simulink model "Filter_Responses"  (R2021a)
settings: Solver=VariableStepAuto  StartTime=0.0  StopTime=3  RelTol=1e-3
libraries: spsCurrentMeasurementLib x4, spsSeriesRLCBranchLib x4, spsVoltageMeasurementLib x4, spsGroundLib x2, spsUniversalBridgeLib x1, spsThreePhaseProgrammableVoltageSourceLib x1, spspowerguiLib x1
settings Model: Creator=Dell  LastModifiedBy=Dell
settings SolverCC: ZeroCrossControl=DisableAll

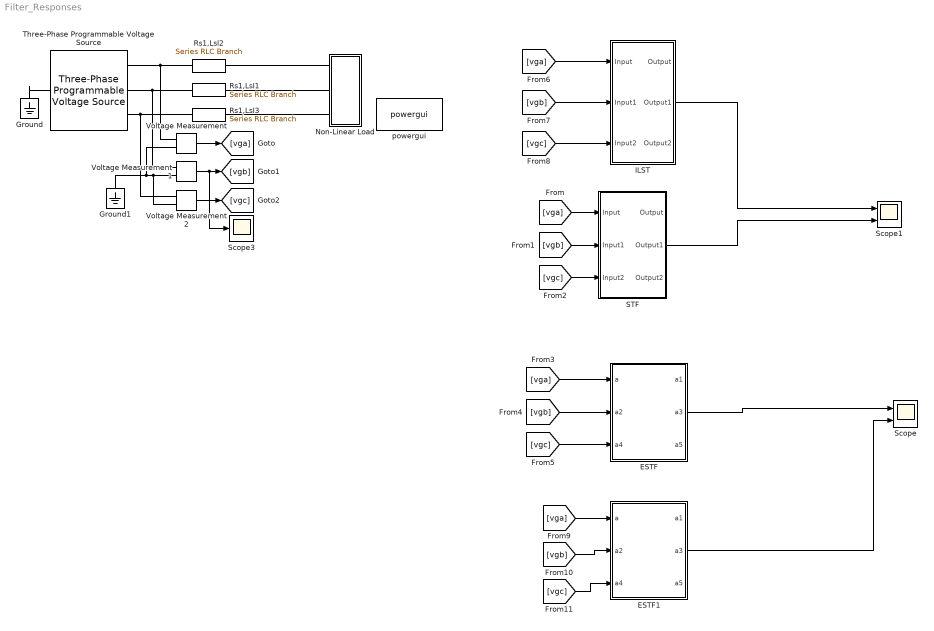
== system Filter_Responses ==
  ESTF : Subsystem
  ESTF1 : Subsystem
  Ground : spsGroundLib/Ground  LConnTagsString=a
  Ground1 : spsGroundLib/Ground  LConnTagsString=a
  ILST : Subsystem
  Non-Linear Load : Subsystem
  Rs1,LsI1 : spsSeriesRLCBranchLib/Series RLC Branch  LConnTagsString=__new0  RConnTagsString=__new0  BranchType=RL  Resistance=.1  Inductance=0.5e-3  SetiL0=off  InitialCurrent=0  Capacitance=1e-6  Setx0=off  InitialVoltage=0  Measurements=None
  Rs1,LsI2 : spsSeriesRLCBranchLib/Series RLC Branch  LConnTagsString=__new0  RConnTagsString=__new0  BranchType=RL  Resistance=.1  Inductance=0.5e-3  SetiL0=off  InitialCurrent=0  Capacitance=1e-6  Setx0=off  InitialVoltage=0  Measurements=None
  Rs1,LsI3 : spsSeriesRLCBranchLib/Series RLC Branch  LConnTagsString=__new0  RConnTagsString=__new0  BranchType=RL  Resistance=.1  Inductance=0.5e-3  SetiL0=off  InitialCurrent=0  Capacitance=1e-6  Setx0=off  InitialVoltage=0  Measurements=None
  STF : Subsystem
  Scope : Scope  NumInputPorts=2
  Scope1 : Scope  NumInputPorts=2
  Scope3 : Scope
  Three-Phase Programmable Voltage Source : spsThreePhaseProgrammableVoltageSourceLib/Three-Phase Programmable Voltage Source  PositiveSequence="[400  0 50]"  VariationEntity=None  VariationType=Table of time-amplitude pairs  VariationTypeAlt=Step  VariationStep=0.5  VariationRate=10  VariationMagnitude=0.3  VariationFrequency=2  VariationTiming=[1 2]  VariationPhaseA=off  Amplitudes=[1 0.8 1.2 1.0]  TimeValues=[0 0.1 0.15 0.2]  HarmonicGeneration=on  HarmonicA=[3 0.02 -25 0]  HarmonicB=[5 0.03 35 2]  Timing="[0.05  3]"  BusType=swing  Pref=0  Qref=0  Qmin=-inf  Qmax=inf
  Voltage Measurement : spsVoltageMeasurementLib/Voltage Measurement  PhasorSimulation=off  OutputType=Complex  PSBequivalent=0
  Voltage Measurement1 : spsVoltageMeasurementLib/Voltage Measurement  PhasorSimulation=off  OutputType=Complex  PSBequivalent=0
  Voltage Measurement2 : spsVoltageMeasurementLib/Voltage Measurement  PhasorSimulation=off  OutputType=Complex  PSBequivalent=0
  powergui : spspowerguiLib/powergui  Priority=1  SimulationMode=Discrete  SampleTime=5e-6  frequency=60  Iterations=50  frequencyindice=50  Pbase=100e6  ErrMax=1e-4  UnitsV=kV  UnitsW=MW  buscounter=0  FunctionMessages=off  echomessages=off  EnableUseOfTLC=off  CurrentSourceSwitches=off  DisableSnubberDevices=off  DisableRonSwitches=off  DisableVfSwitches=off  DisplayEquations=off  AutomaticDiscreteSolvers=off  SolverType=Tustin/Backward Euler (TBE)  Interpol=off  ExternalGateDelay=off  methode=off  Ts=100  x0status=blocks  SPID=on  SwTol=0  HookPort=off  NonlinearTolerance=1e-4  nMaxIteration=100  ContinueOnMaxIteration=off  RestoreLinks=warning  ResistiveCurrentMeasurement=off  Frange=[0:2:500]  Ylog=off  Xlog=on  ShowGrid=off  save=off  variable=ZData  structure=0  ZoomFFT=off  StartTime=0.0  cycles=1  DisplayStyle=1  fundamental=60  FreqAxis=off  MaxFrequency=1000  frequencyindicesteady=1  RmsSteady=1  display=off
  wires:
  Voltage Measurement/1 -> [vga]
  Voltage Measurement1/1 -> Scope3/1, [vgb]
  Voltage Measurement2/1 -> [vgc]
  [vga] -> STF/1(Input)
  [vgb] -> STF/2(Input1)
  [vgc] -> STF/3(Input2)
  [vgc] -> ESTF/3(a4)
  [vga] -> ESTF/1(a)
  [vgb] -> ESTF/2(a2)
  [vgc] -> ILST/3(Input2)
  [vga] -> ILST/1(Input)
  [vgb] -> ILST/2(Input1)
  ILST/2(Output1) -> Scope1/1
  STF/2(Output1) -> Scope1/2
  ESTF/2(a3) -> Scope/1
  [vga] -> ESTF1/1(a)
  [vgb] -> ESTF1/2(a2)
  [vgc] -> ESTF1/3(a4)
  ESTF1/2(a3) -> Scope/2
  connections:
  Three-Phase Programmable Voltage Source/RConn3 -- Voltage Measurement2/LConn1 -- Rs1,LsI3/LConn1
  Rs1,LsI1/LConn1 -- Voltage Measurement1/LConn1 -- Three-Phase Programmable Voltage Source/RConn2
  Rs1,LsI2/LConn1 -- Voltage Measurement/LConn1 -- Three-Phase Programmable Voltage Source/RConn1
  Rs1,LsI2/RConn1 -- Non-Linear Load/LConn1
  Rs1,LsI1/RConn1 -- Non-Linear Load/LConn2
  Rs1,LsI3/RConn1 -- Non-Linear Load/LConn3
  Ground/LConn1 -- Three-Phase Programmable Voltage Source/LConn1
  Ground1/LConn1 -- Voltage Measurement2/LConn2 -- Voltage Measurement1/LConn2 -- Voltage Measurement/LConn2

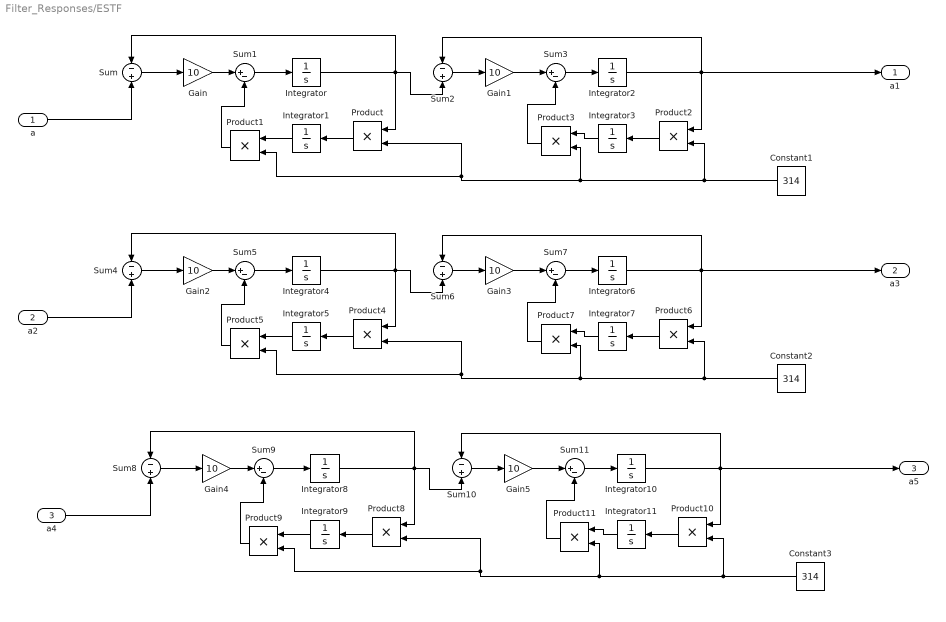
== system Filter_Responses/ESTF ==
  a : Inport
  a2 : Inport  Port=2
  a4 : Inport  Port=3
  Constant1 : Constant  Value=314
  Constant2 : Constant  Value=314
  Constant3 : Constant  Value=314
  Gain{,1..5} (6 alike) : Gain  Gain=10
  Integrator{,1..11} (12 alike) : Integrator
  Product{,1..11} (12 alike) : Product
  Sum{,2,4,6,8,10} (6 alike) : Sum  Inputs=-+
  Sum{1,3,5,7,9,11} (6 alike) : Sum  Inputs=|+-
  a1 : Outport
  a3 : Outport  Port=2
  a5 : Outport  Port=3
  wires:
  Sum/1 -> Gain/1
  Integrator/1 -> Sum/1, Sum2/2, Product/1
  Product3/1 -> Sum3/2
  Product1/1 -> Sum1/2
  Product2/1 -> Integrator3/1
  Constant1/1 -> Product2/2, Product3/2, Product1/2, Product/2
  Integrator2/1 -> a1/1, Product2/1, Sum2/1
  Integrator1/1 -> Product1/1
  Gain1/1 -> Sum3/1
  Sum3/1 -> Integrator2/1
  a/1 -> Sum/2
  Gain/1 -> Sum1/1
  Product/1 -> Integrator1/1
  Sum1/1 -> Integrator/1
  Sum2/1 -> Gain1/1
  Integrator3/1 -> Product3/1
  Gain3/1 -> Sum7/1
  Sum7/1 -> Integrator6/1
  Sum6/1 -> Gain3/1
  Product6/1 -> Integrator7/1
  a2/1 -> Sum4/2
  Product5/1 -> Sum5/2
  Integrator7/1 -> Product7/1
  Gain2/1 -> Sum5/1
  Constant2/1 -> Product6/2, Product7/2, Product5/2, Product4/2
  Sum5/1 -> Integrator4/1
  Product4/1 -> Integrator5/1
  Integrator5/1 -> Product5/1
  Product7/1 -> Sum7/2
  Integrator4/1 -> Sum4/1, Sum6/2, Product4/1
  Sum4/1 -> Gain2/1
  Integrator6/1 -> a3/1, Product6/1, Sum6/1
  Gain5/1 -> Sum11/1
  Sum11/1 -> Integrator10/1
  Sum10/1 -> Gain5/1
  Product10/1 -> Integrator11/1
  a4/1 -> Sum8/2
  Product9/1 -> Sum9/2
  Integrator11/1 -> Product11/1
  Gain4/1 -> Sum9/1
  Constant3/1 -> Product10/2, Product11/2, Product9/2, Product8/2
  Sum9/1 -> Integrator8/1
  Product8/1 -> Integrator9/1
  Integrator9/1 -> Product9/1
  Product11/1 -> Sum11/2
  Integrator8/1 -> Sum8/1, Sum10/2, Product8/1
  Sum8/1 -> Gain4/1
  Integrator10/1 -> a5/1, Product10/1, Sum10/1

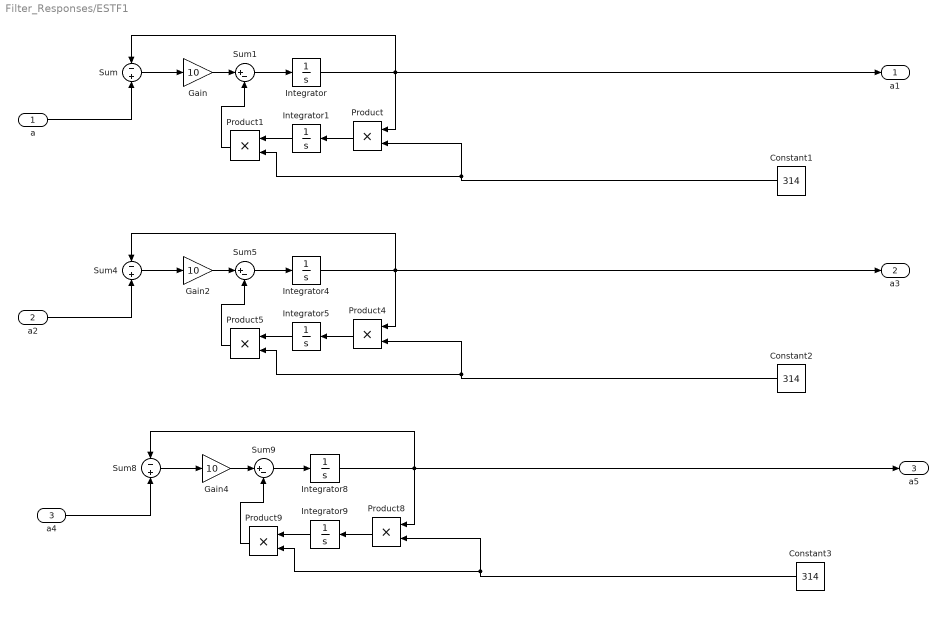
== system Filter_Responses/ESTF1 ==
  a : Inport
  a2 : Inport  Port=2
  a4 : Inport  Port=3
  Constant1 : Constant  Value=314
  Constant2 : Constant  Value=314
  Constant3 : Constant  Value=314
  Gain : Gain  Gain=10
  Gain2 : Gain  Gain=10
  Gain4 : Gain  Gain=10
  Integrator{,1,4..5,8..9} (6 alike) : Integrator
  Product{,1,4..5,8..9} (6 alike) : Product
  Sum : Sum  Inputs=-+
  Sum1 : Sum  Inputs=|+-
  Sum4 : Sum  Inputs=-+
  Sum5 : Sum  Inputs=|+-
  Sum8 : Sum  Inputs=-+
  Sum9 : Sum  Inputs=|+-
  a1 : Outport
  a3 : Outport  Port=2
  a5 : Outport  Port=3
  wires:
  Sum/1 -> Gain/1
  Integrator/1 -> a1/1, Sum/1, Product/1
  Product1/1 -> Sum1/2
  Constant1/1 -> Product1/2, Product/2
  Integrator1/1 -> Product1/1
  a/1 -> Sum/2
  Gain/1 -> Sum1/1
  Product/1 -> Integrator1/1
  Sum1/1 -> Integrator/1
  a2/1 -> Sum4/2
  Product5/1 -> Sum5/2
  Gain2/1 -> Sum5/1
  Constant2/1 -> Product5/2, Product4/2
  Sum5/1 -> Integrator4/1
  Product4/1 -> Integrator5/1
  Integrator5/1 -> Product5/1
  Integrator4/1 -> a3/1, Sum4/1, Product4/1
  Sum4/1 -> Gain2/1
  a4/1 -> Sum8/2
  Product9/1 -> Sum9/2
  Gain4/1 -> Sum9/1
  Constant3/1 -> Product9/2, Product8/2
  Sum9/1 -> Integrator8/1
  Product8/1 -> Integrator9/1
  Integrator9/1 -> Product9/1
  Integrator8/1 -> a5/1, Sum8/1, Product8/1
  Sum8/1 -> Gain4/1

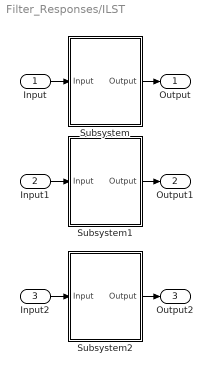
== system Filter_Responses/ILST ==
  Input : Inport
  Input1 : Inport  Port=2
  Input2 : Inport  Port=3
  Subsystem : Subsystem
  Subsystem1 : Subsystem
  Subsystem2 : Subsystem
  Output : Outport
  Output1 : Outport  Port=2
  Output2 : Outport  Port=3
  wires:
  Input2/1 -> Subsystem2/1(Input)
  Subsystem2/1(Output) -> Output2/1
  Subsystem/1(Output) -> Output/1
  Input/1 -> Subsystem/1(Input)
  Input1/1 -> Subsystem1/1(Input)
  Subsystem1/1(Output) -> Output1/1

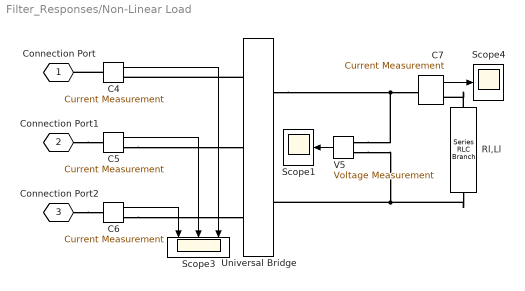
== system Filter_Responses/Non-Linear Load ==
  C{4..7} (4 alike) : spsCurrentMeasurementLib/Current Measurement  PhasorSimulation=off  OutputType=Complex  PSBequivalent=0
  Rl,Ll : spsSeriesRLCBranchLib/Series RLC Branch  LConnTagsString=__new0  RConnTagsString=__new0  BranchType=RL  Resistance=200  Inductance=25e-3  SetiL0=off  InitialCurrent=0  Capacitance=1.0  Setx0=off  InitialVoltage=0  Measurements=None
  Scope1 : Scope
  Scope3 : Scope  NumInputPorts=3
  Scope4 : Scope
  Universal Bridge : spsUniversalBridgeLib/Universal Bridge  Arms=3  SnubberResistance=500  SnubberCapacitance=.1e-6  Device=Diodes  Ron=1e-3  Lon=0  ForwardVoltages="[  0  0  ]"  ForwardVoltage=.8  GTOparameters=[ 10e-6 , 20e-6 ]  IGBTparameters=[ 1e-6 , 2e-6 ]  Measurements=Device voltages  Measurements_2=None  converterType=Rectifier
  V5 : spsVoltageMeasurementLib/Voltage Measurement  PhasorSimulation=off  OutputType=Complex  PSBequivalent=0
  Connection Port : PMIOPort  Tag=PMCPort  Side=Left
  Connection Port1 : PMIOPort  Tag=PMCPort  Port=2  Side=Left
  Connection Port2 : PMIOPort  Tag=PMCPort  Port=3  Side=Left
  wires:
  C7/1 -> Scope4/1
  V5/1 -> Scope1/1
  C6/1 -> Scope3/1
  C5/1 -> Scope3/2
  C4/1 -> Scope3/3
  connections:
  Universal Bridge/RConn1 -- V5/LConn1 -- C7/LConn1
  Rl,Ll/LConn1 -- C7/RConn1
  Rl,Ll/RConn1 -- V5/LConn2 -- Universal Bridge/RConn2
  C4/LConn1 -- Connection Port/RConn1
  Connection Port2/RConn1 -- C6/LConn1
  Connection Port1/RConn1 -- C5/LConn1
  C6/RConn1 -- Universal Bridge/LConn3
  C5/RConn1 -- Universal Bridge/LConn2
  Universal Bridge/LConn1 -- C4/RConn1

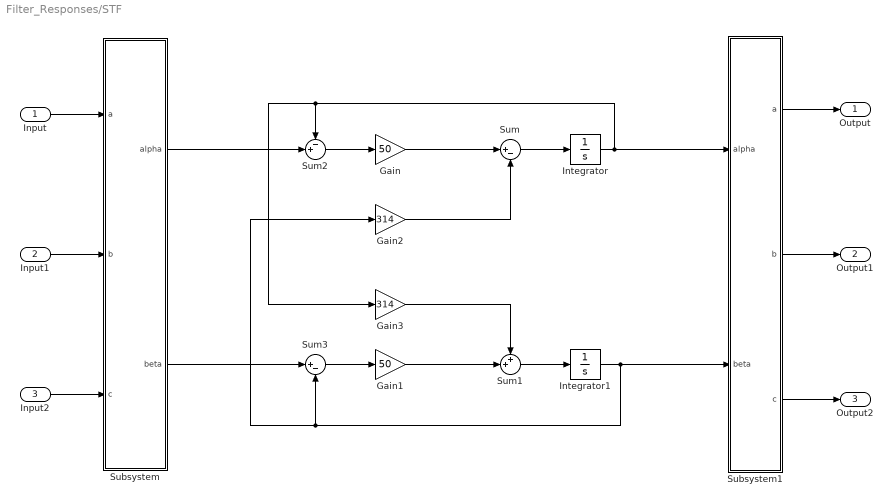
== system Filter_Responses/STF ==
  Input : Inport
  Input1 : Inport  Port=2
  Input2 : Inport  Port=3
  Gain : Gain  Gain=50
  Gain1 : Gain  Gain=50
  Gain2 : Gain  Gain=314
  Gain3 : Gain  Gain=314
  Integrator : Integrator
  Integrator1 : Integrator
  Subsystem : Subsystem
  Subsystem1 : Subsystem
  Sum : Sum  Inputs=|+-
  Sum1 : Sum  Inputs=++|
  Sum2 : Sum  Inputs=-+|
  Sum3 : Sum  Inputs=|+-
  Output : Outport
  Output1 : Outport  Port=2
  Output2 : Outport  Port=3
  wires:
  Subsystem1/2(b) -> Output1/1
  Gain3/1 -> Sum1/1
  Input/1 -> Subsystem/1(a)
  Input2/1 -> Subsystem/3(c)
  Input1/1 -> Subsystem/2(b)
  Gain1/1 -> Sum1/2
  Subsystem1/1(a) -> Output/1
  Integrator1/1 -> Sum3/2, Gain2/1, Subsystem1/2(beta)
  Sum2/1 -> Gain/1
  Subsystem/1(alpha) -> Sum2/2
  Sum1/1 -> Integrator1/1
  Sum/1 -> Integrator/1
  Gain/1 -> Sum/1
  Subsystem1/3(c) -> Output2/1
  Integrator/1 -> Sum2/1, Gain3/1, Subsystem1/1(alpha)
  Gain2/1 -> Sum/2
  Sum3/1 -> Gain1/1
  Subsystem/2(beta) -> Sum3/1

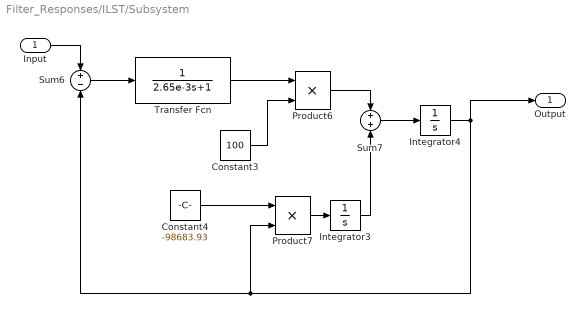
== system Filter_Responses/ILST/Subsystem ==
  Input : Inport
  Constant3 : Constant  Value=100
  Constant4 : Constant  Value=-98683.93
  Integrator3 : Integrator
  Integrator4 : Integrator
  Product6 : Product  RndMeth=Zero
  Product7 : Product  RndMeth=Zero
  Sum6 : Sum  Inputs=+-
  Sum7 : Sum
  Transfer Fcn : TransferFcn  Denominator=[2.65e-3 1]
  Output : Outport
  wires:
  Sum6/1 -> Transfer Fcn/1
  Product6/1 -> Sum7/1
  Input/1 -> Sum6/1
  Integrator4/1 -> Output/1, Product7/2, Sum6/2
  Constant3/1 -> Product6/2
  Constant4/1 -> Product7/1
  Sum7/1 -> Integrator4/1
  Transfer Fcn/1 -> Product6/1
  Product7/1 -> Integrator3/1
  Integrator3/1 -> Sum7/2

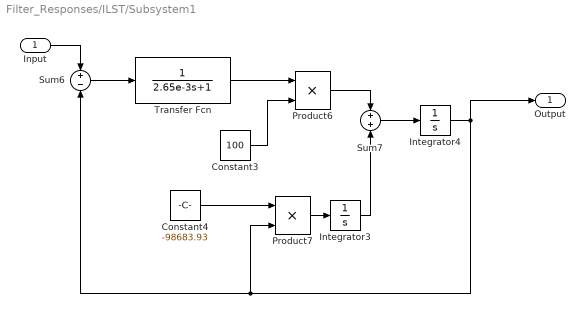
== system Filter_Responses/ILST/Subsystem1 ==
  Input : Inport
  Constant3 : Constant  Value=100
  Constant4 : Constant  Value=-98683.93
  Integrator3 : Integrator
  Integrator4 : Integrator
  Product6 : Product  RndMeth=Zero
  Product7 : Product  RndMeth=Zero
  Sum6 : Sum  Inputs=+-
  Sum7 : Sum
  Transfer Fcn : TransferFcn  Denominator=[2.65e-3 1]
  Output : Outport
  wires:
  Sum6/1 -> Transfer Fcn/1
  Product6/1 -> Sum7/1
  Input/1 -> Sum6/1
  Integrator4/1 -> Output/1, Product7/2, Sum6/2
  Constant3/1 -> Product6/2
  Constant4/1 -> Product7/1
  Sum7/1 -> Integrator4/1
  Transfer Fcn/1 -> Product6/1
  Product7/1 -> Integrator3/1
  Integrator3/1 -> Sum7/2

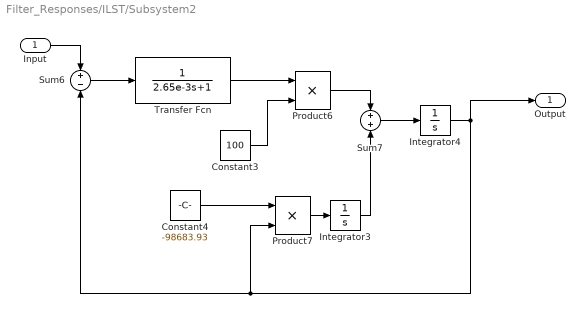
== system Filter_Responses/ILST/Subsystem2 ==
  Input : Inport
  Constant3 : Constant  Value=100
  Constant4 : Constant  Value=-98683.93
  Integrator3 : Integrator
  Integrator4 : Integrator
  Product6 : Product  RndMeth=Zero
  Product7 : Product  RndMeth=Zero
  Sum6 : Sum  Inputs=+-
  Sum7 : Sum
  Transfer Fcn : TransferFcn  Denominator=[2.65e-3 1]
  Output : Outport
  wires:
  Sum6/1 -> Transfer Fcn/1
  Product6/1 -> Sum7/1
  Input/1 -> Sum6/1
  Integrator4/1 -> Output/1, Product7/2, Sum6/2
  Constant3/1 -> Product6/2
  Constant4/1 -> Product7/1
  Sum7/1 -> Integrator4/1
  Transfer Fcn/1 -> Product6/1
  Product7/1 -> Integrator3/1
  Integrator3/1 -> Sum7/2

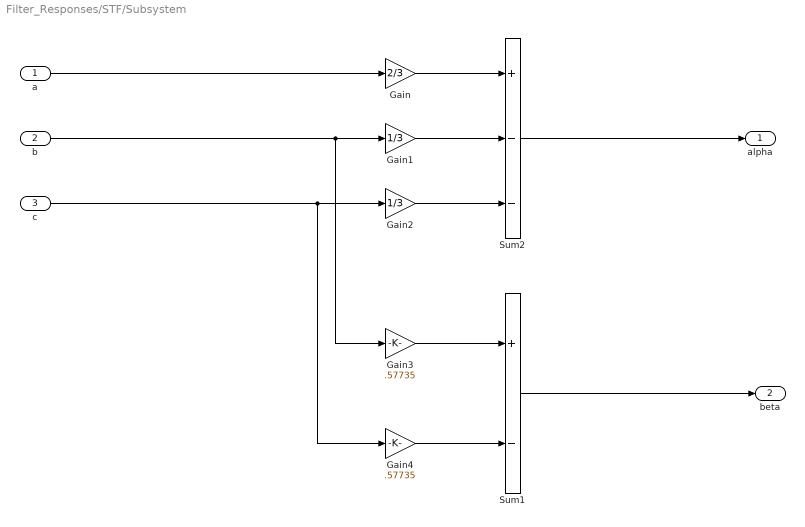
== system Filter_Responses/STF/Subsystem ==
  a : Inport
  b : Inport  Port=2
  c : Inport  Port=3
  Gain : Gain  Gain=2/3
  Gain1 : Gain  Gain=1/3
  Gain2 : Gain  Gain=1/3
  Gain3 : Gain  Gain=.57735
  Gain4 : Gain  Gain=.57735
  Sum1 : Sum  Inputs=+-
  Sum2 : Sum  Inputs=+--
  alpha : Outport
  beta : Outport  Port=2
  wires:
  Gain/1 -> Sum2/1
  Gain1/1 -> Sum2/2
  Gain2/1 -> Sum2/3
  Sum2/1 -> alpha/1
  a/1 -> Gain/1
  b/1 -> Gain3/1, Gain1/1
  c/1 -> Gain4/1, Gain2/1
  Sum1/1 -> beta/1
  Gain4/1 -> Sum1/2
  Gain3/1 -> Sum1/1

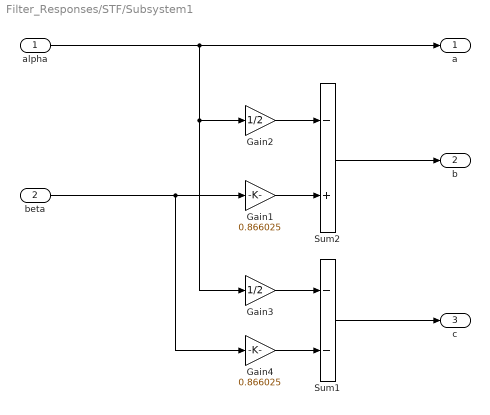
== system Filter_Responses/STF/Subsystem1 ==
  alpha : Inport
  beta : Inport  Port=2
  Gain1 : Gain  Gain=0.866025
  Gain2 : Gain  Gain=1/2
  Gain3 : Gain  Gain=1/2
  Gain4 : Gain  Gain=0.866025
  Sum1 : Sum  Inputs=--
  Sum2 : Sum  Inputs=-+
  a : Outport
  b : Outport  Port=2
  c : Outport  Port=3
  wires:
  Gain3/1 -> Sum1/1
  Gain4/1 -> Sum1/2
  Sum1/1 -> c/1
  alpha/1 -> a/1, Gain3/1, Gain2/1
  Gain2/1 -> Sum2/1
  Gain1/1 -> Sum2/2
  Sum2/1 -> b/1
  beta/1 -> Gain4/1, Gain1/1
